simulink library "Mix_T_Mdot"  (Simulink 8.2)
settings: Solver=ode45  StartTime=0.0  StopTime=10.0  RelTol=1e-3
settings Model: Creator=lena.frank  LastModifiedBy=drhf

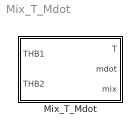
== system Mix_T_Mdot ==
  Mix_T_Mdot : Subsystem  mask(mix_temperature){mixcalc=Tmix = (mdot1*T1 + mdot2*T2)/(mdot1+mdot2)}
      mask prompts: mixcalc "Calculation of mixture :"
      mask help:
      | Calculate the temperature of the mixture of two flows. Uses enthalpy balance for humid air. Liquids may be mixed by the (faster and approximate) equation:
      | Tmix = (mdot1*T1 + mdot2*T2)/(mdot1+mdot2)
      mask Help: web(fullfile(path_carnot('help'),'Mix_T_Mdot.html'),'-helpbrowser')
      mask TypeOptions mixcalc: Tmix = (mdot1*T1 + mdot2*T2)/(mdot1+mdot2) | Enthalpy balance

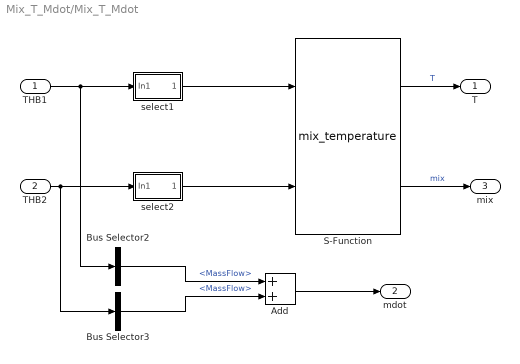
== system Mix_T_Mdot/Mix_T_Mdot ==
  THB1 : Inport
  THB2 : Inport  Port=2
  Add : Sum
  Bus Selector2 : BusSelector  OutputSignals=MassFlow
  Bus Selector3 : BusSelector  OutputSignals=MassFlow
  S-Function : S-Function  FunctionName=mix_temperature  Parameters=mixcalc  EnableBusSupport=off
  select1 : Subsystem
  select2 : Subsystem
  T : Outport
  mdot : Outport  Port=2
  mix : Outport  Port=3
  wires:
  Add/1 -> mdot/1
  Bus Selector2/1 -> Add/1  "<MassFlow>"
  Bus Selector3/1 -> Add/2  "<MassFlow>"
  THB1/1 -> Bus Selector2/1, select1/1(In1)
  S-Function/2 -> mix/1  "mix"
  THB2/1 -> Bus Selector3/1, select2/1(In1)
  S-Function/1 -> T/1  "T"
  select1/1(Out1) -> S-Function/1
  select2/1(Out1) -> S-Function/2

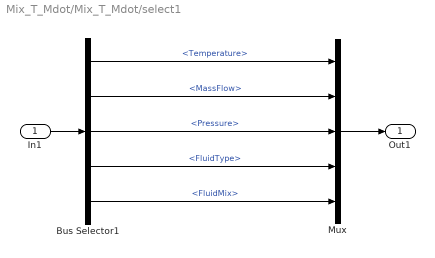
== system Mix_T_Mdot/Mix_T_Mdot/select1 ==
  In1 : Inport
  Bus Selector1 : BusSelector  OutputSignals=Temperature,MassFlow,Pressure,FluidType,FluidMix
  Mux : Mux  Inputs=5
  Out1 : Outport
  wires:
  Bus Selector1/1 -> Mux/1  "<Temperature>"
  Bus Selector1/2 -> Mux/2  "<MassFlow>"
  Bus Selector1/3 -> Mux/3  "<Pressure>"
  Bus Selector1/4 -> Mux/4  "<FluidType>"
  Bus Selector1/5 -> Mux/5  "<FluidMix>"
  In1/1 -> Bus Selector1/1
  Mux/1 -> Out1/1

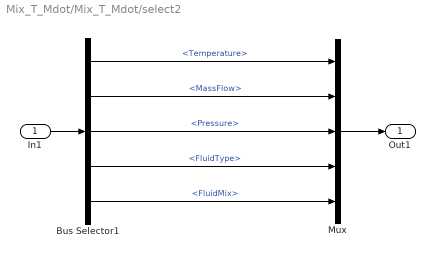
== system Mix_T_Mdot/Mix_T_Mdot/select2 ==
  In1 : Inport
  Bus Selector1 : BusSelector  OutputSignals=Temperature,MassFlow,Pressure,FluidType,FluidMix
  Mux : Mux  Inputs=5
  Out1 : Outport
  wires:
  Mux/1 -> Out1/1
  In1/1 -> Bus Selector1/1
  Bus Selector1/5 -> Mux/5  "<FluidMix>"
  Bus Selector1/4 -> Mux/4  "<FluidType>"
  Bus Selector1/3 -> Mux/3  "<Pressure>"
  Bus Selector1/2 -> Mux/2  "<MassFlow>"
  Bus Selector1/1 -> Mux/1  "<Temperature>"
